simulink model "simulink_ft_fault_injection"  (R2020b)
settings: Solver=FixedStepAuto  StartTime=0.0  StopTime=Tend  FixedStep=hp  RelTol=1e-3
undefined symbols (not defined in the file): Ad_plant, Bd_plant, controller_mode, delay_length, error_probability, f, F_total, hp, K_total, mode_switching_enable, n, ref, ref_array, ref_enable, ref_sampling_factor, Sat_u, Sm
settings Model: SimulationMode=accelerator  SnapshotInterval=2  Creator=juan  LastModifiedBy=jvalencia
settings DataIOCC: ReturnWorkspaceOutputs=off
settings DebuggingCC: ArithmeticOperatorsInVariantConditions=warning
settings SFSimCC: SimUseLocalCustomCode=off  CustomCodeUndefinedFunction=UseInterfaceOnly
settings RTWCC: RTWUseLocalCustomCode=off
settings CodeAppCC: StateflowObjectComments=on

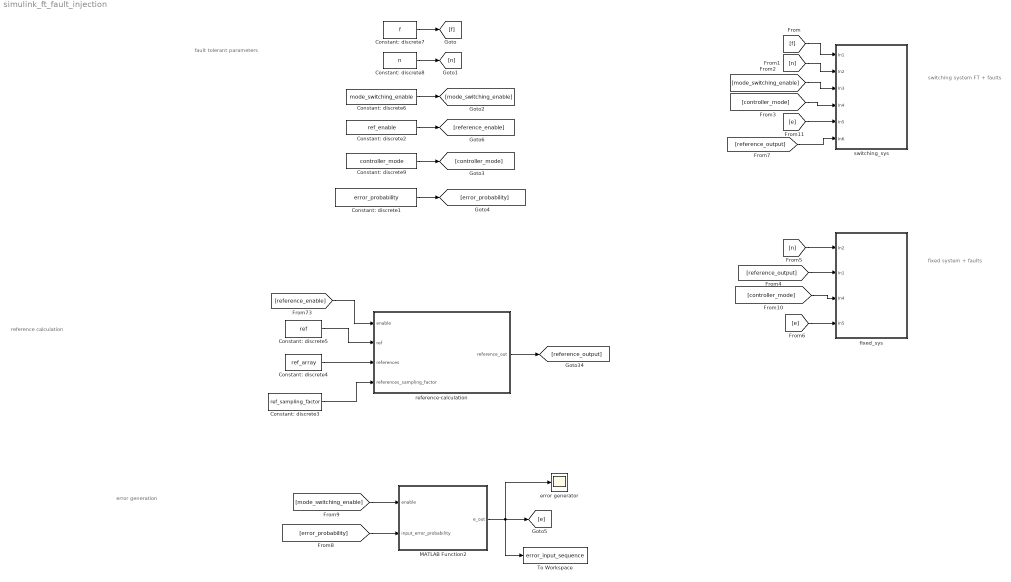
== system simulink_ft_fault_injection ==
  note: fault tolerant parameters
  note: switching system FT + faults
  note: error generation
  note: fixed system + faults
  note: reference calculation
  Constant: discrete1 : Constant  Value=error_probability  SampleTime=Sm
  Constant: discrete2 : Constant  Value=ref_enable  SampleTime=Sm
  Constant: discrete3 : Constant  Value=ref_sampling_factor  OutDataTypeStr=single  SampleTime=Sm
  Constant: discrete4 : Constant  Value=ref_array  OutDataTypeStr=single  SampleTime=Sm
  Constant: discrete5 : Constant  Value=ref  OutDataTypeStr=single  SampleTime=Sm
  Constant: discrete6 : Constant  Value=mode_switching_enable  SampleTime=Sm
  Constant: discrete7 : Constant  Value=f  OutDataTypeStr=single  SampleTime=Sm
  Constant: discrete8 : Constant  Value=n  OutDataTypeStr=single  SampleTime=Sm
  Constant: discrete9 : Constant  Value=controller_mode  SampleTime=Sm
  MATLAB Function2 : MATLAB Function  TreatAsAtomicUnit=on  SystemSampleTime=Sm
  To Workspace : ToWorkspace  VariableName=error_input_sequence  SaveFormat=Timeseries  SampleTime=Sm
  "error generator " : Scope
  fixed_sys : Subsystem
  reference-calculation : MATLAB Function  TreatAsAtomicUnit=on
  switching_sys : Subsystem
  wires:
  Constant: discrete7/1 -> [f]
  Constant: discrete8/1 -> [n]
  Constant: discrete6/1 -> [mode_switching_enable]
  Constant: discrete9/1 -> [controller_mode]
  [f] -> switching_sys/1(In1)
  [n] -> switching_sys/2(In2)
  [mode_switching_enable] -> switching_sys/3(In3)
  [controller_mode] -> switching_sys/4(In4)
  Constant: discrete1/1 -> [error_probability]
  [mode_switching_enable] -> MATLAB Function2/1(enable)
  [error_probability] -> MATLAB Function2/2(input_error_probability)
  MATLAB Function2/1(e_out) -> "error generator "/1, To Workspace/1, [e]
  [e] -> switching_sys/5(In5)
  [n] -> fixed_sys/1(In2)
  [controller_mode] -> fixed_sys/3(In4)
  [e] -> fixed_sys/4(In5)
  Constant: discrete2/1 -> [reference_enable]
  Constant: discrete4/1 -> reference-calculation/3(references)
  reference-calculation/1(reference_out) -> [reference_output]
  Constant: discrete3/1 -> reference-calculation/4(references_sampling_factor)
  Constant: discrete5/1 -> reference-calculation/2(ref)
  [reference_enable] -> reference-calculation/1(enable)
  [reference_output] -> fixed_sys/2(In1)
  [reference_output] -> switching_sys/6(In6)

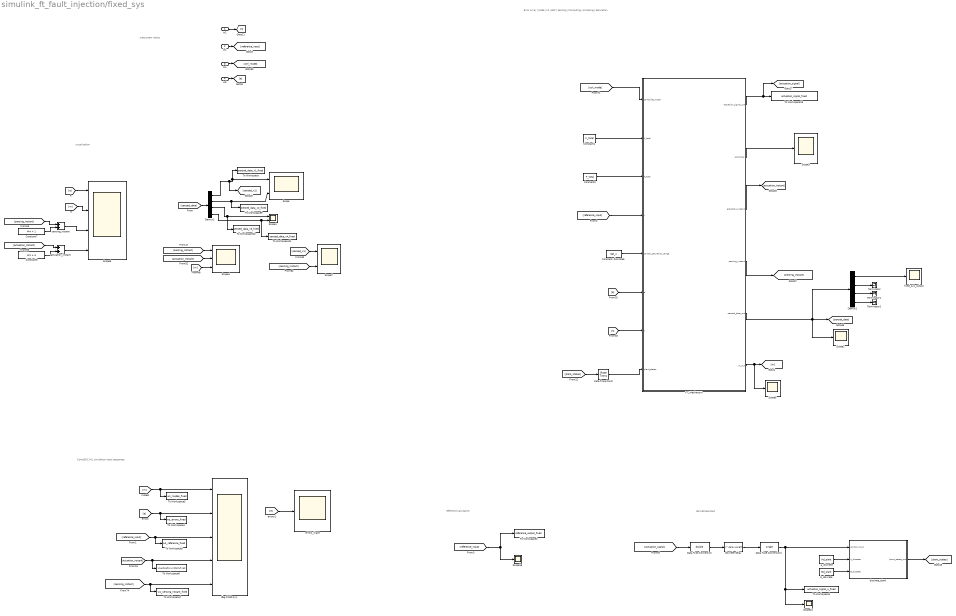
== system simulink_ft_fault_injection/fixed_sys ==
  note: Error Array | Mode | LC | EFC |
      | Sensing | Computing | Actuating | Saturation
  note: discretized plant
  note: reference calculation
  note: subsystem inputs
  note: CompSOC HIL simulation input sequences
  note: visualization
  In2 : Inport
  In1 : Inport  Port=2
  In4 : Inport  Port=3
  In5 : Inport  Port=4
  Constant1 : Constant  Value=K_total  OutDataTypeStr=single  SampleTime=Sm
  Constant2 : Constant  Value=F_total  OutDataTypeStr=single  SampleTime=Sm
  Constant7 : Constant  Value=4*n + 1  SampleTime=Sm
  Constant9 : Constant  Value=4*n + 3  SampleTime=Sm
  Constant: discrete6 : Constant  Value=Sat_u  OutDataTypeStr=single  SampleTime=Sm
  Data Type Conversion : DataTypeConversion  OutDataTypeStr=double
  Data Type Conversion1 : DataTypeConversion  OutDataTypeStr=single
  Demux1 : Demux
  Demux2 : Demux
  FT_mechanism : MATLAB Function  TreatAsAtomicUnit=on
  Rate Transition2 : RateTransition  OutPortSampleTime=Sm
  Scope : Scope  NumInputPorts=2
  Scope1 : Scope  NumInputPorts=2
  Scope{2..3,5,10,16} (5 alike) : Scope
  Scope4 : Scope  NumInputPorts=3
  Scope7 : Scope  NumInputPorts=2
  Scope9 : Scope  NumInputPorts=4
  Terminator : Terminator
  Terminator1 : Terminator
  Terminator2 : Terminator
  To Workspace : ToWorkspace  VariableName=sensed_data_x1_fixed  SaveFormat=Timeseries  SampleTime=Sm
  To Workspace1 : ToWorkspace  VariableName=actuation_signal_u_fixed  SaveFormat=Timeseries  SampleTime=Sm
  To Workspace10 : ToWorkspace  VariableName=sensed_data_x3_fixed  SaveFormat=Timeseries  SampleTime=Sm
  To Workspace11 : ToWorkspace  VariableName=sensed_data_x4_fixed  SaveFormat=Timeseries  SampleTime=Sm
  To Workspace13 : ToWorkspace  VariableName=actuation_signal_fixed  SaveFormat=Timeseries  SampleTime=Sm
  To Workspace2 : ToWorkspace  VariableName=reference_output_fixed  SaveFormat=Timeseries  SampleTime=Sm
  To Workspace3 : ToWorkspace  VariableName=ws_modes_fixed  SaveFormat=Timeseries  SampleTime=Sm
  To Workspace4 : ToWorkspace  VariableName=ws_errors_fixed  SaveFormat=Timeseries  SampleTime=Sm
  To Workspace5 : ToWorkspace  VariableName=ws_reference_fixed  SaveFormat=Timeseries  SampleTime=Sm
  To Workspace6 : ToWorkspace  VariableName=ws_actuation_instant_fixed  SaveFormat=Timeseries  SampleTime=Sm
  To Workspace7 : ToWorkspace  VariableName=ws_sensing_instant_fixed  SaveFormat=Timeseries  SampleTime=Sm
  To Workspace9 : ToWorkspace  VariableName=sensed_data_x2_fixed  SaveFormat=Timeseries  SampleTime=Sm
  a_discrete : Constant  Value=Ad_plant  OutDataTypeStr=single  SampleTime=hp
  actuation_instant : Sum
  b_discrete : Constant  Value=Bd_plant  OutDataTypeStr=single  SampleTime=hp
  dbg FIXED sys. : Scope  NumInputPorts=5
  discrete-delay : Delay  DelayLength=delay_length  SampleTime=hp
  discrete_plant : MATLAB Function  TreatAsAtomicUnit=on  SystemSampleTime=hp
  errors_trace : Scope
  "fixed_sys_output " : Scope
  sensing_instant : Sum
  wires:
  [reference_input] -> FT_mechanism/4(r)
  Demux2/1 -> [sensed_x1], To Workspace/1, Scope/1
  actuation_instant/1 -> Scope9/4
  [sensed_x1] -> Scope7/1
  discrete-delay/1 -> Data Type Conversion1/1
  [sensing_instant] -> Scope7/2
  Data Type Conversion/1 -> discrete-delay/1
  [e] -> Scope9/1
  [actuation_signal] -> Data Type Conversion/1
  [reference_input] -> To Workspace2/1, Scope16/1
  Data Type Conversion1/1 -> discrete_plant/1(control_input), To Workspace1/1, Scope10/1
  Demux2/3 -> To Workspace10/1, Scope1/1
  Demux2/4 -> To Workspace11/1, Scope1/2
  Demux2/2 -> To Workspace9/1, Scope/2
  FT_mechanism/1(actuation_signal_out) -> To Workspace13/1, [actuation_signal]
  Constant7/1 -> sensing_instant/2
  FT_mechanism/2(controller) -> Scope3/1
  [actuation_instant] -> actuation_instant/1
  Constant9/1 -> actuation_instant/2
  [sensing_instant] -> sensing_instant/1
  [actuation_instant] -> Scope4/2
  [m] -> Scope4/3
  [sensing_instant] -> Scope4/1
  [m] -> Scope9/2
  [sensed_data] -> Demux2/1
  In2/1 -> [n]
  In4/1 -> [ctrl_mode]
  In5/1 -> [e]
  [m] -> To Workspace3/1, dbg FIXED sys./1
  [reference_input] -> dbg FIXED sys./3, To Workspace5/1
  [e] -> To Workspace4/1, dbg FIXED sys./2
  [actuation_instant] -> To Workspace6/1, dbg FIXED sys./4
  [sensing_instant] -> To Workspace7/1, dbg FIXED sys./5
  a_discrete/1 -> discrete_plant/2(A_discrete)
  b_discrete/1 -> discrete_plant/3(B_discrete)
  discrete_plant/1(plant_states_out) -> [plant_states]
  Constant: discrete6/1 -> FT_mechanism/5(control_saturation_range)
  FT_mechanism/3(actuation_instant) -> [actuation_instant]
  [n] -> FT_mechanism/7(n)
  [e] -> FT_mechanism/6(e)
  Rate Transition2/1 -> FT_mechanism/8(plant_states)
  [plant_states] -> Rate Transition2/1
  FT_mechanism/5(sensed_data_out) -> Demux1/1, Scope2/1, [sensed_data]
  FT_mechanism/4(sensing_instant) -> [sensing_instant]
  [ctrl_mode] -> FT_mechanism/1(controller_mode)
  FT_mechanism/6(m_out) -> Scope5/1, [m]
  [e] -> errors_trace/1
  Demux1/1 -> "fixed_sys_output "/1
  In1/1 -> [reference_input]
  Constant1/1 -> FT_mechanism/2(K_total)
  Constant2/1 -> FT_mechanism/3(F_total)
  Demux1/2 -> Terminator/1
  Demux1/3 -> Terminator1/1
  Demux1/4 -> Terminator2/1
  sensing_instant/1 -> Scope9/3

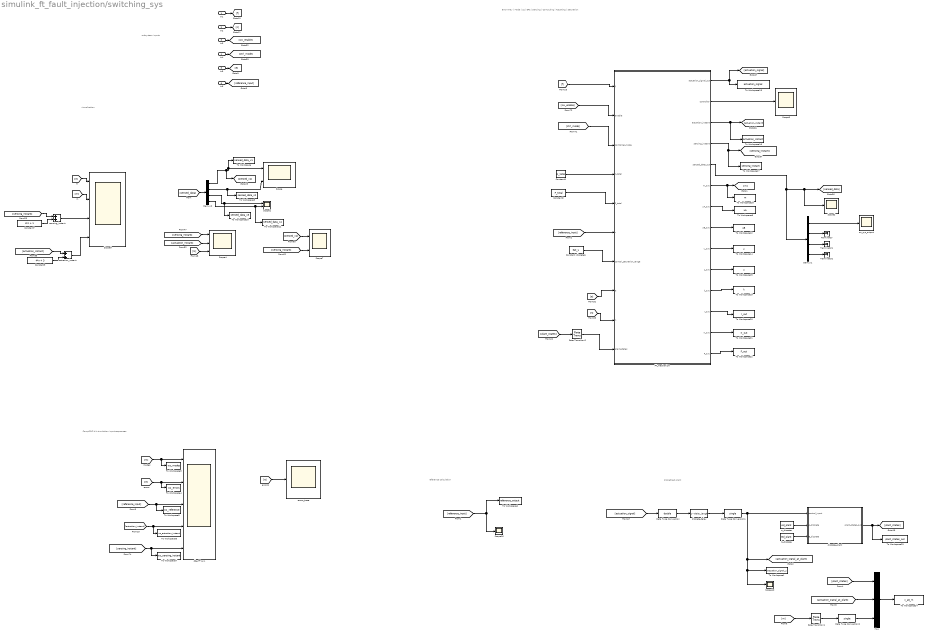
== system simulink_ft_fault_injection/switching_sys ==
  note: Error Array | Mode | LC | EFC |
      | Sensing | Computing | Actuating | Saturation
  note: discretized plant
  note: reference calculation
  note: subsystem inputs
  note: CompSOC HIL simulation input sequences
  note: visualization
  In1 : Inport
  In2 : Inport  Port=2
  In3 : Inport  Port=3
  In4 : Inport  Port=4
  In5 : Inport  Port=5
  In6 : Inport  Port=6
  Constant1 : Constant  Value=K_total  OutDataTypeStr=single  SampleTime=Sm
  Constant2 : Constant  Value=F_total  OutDataTypeStr=single  SampleTime=Sm
  Constant7 : Constant  Value=4*n + 1  SampleTime=Sm
  Constant9 : Constant  Value=4*n + 3  SampleTime=Sm
  Constant: discrete6 : Constant  Value=Sat_u  OutDataTypeStr=single  SampleTime=Sm
  Data Type Conversion : DataTypeConversion  OutDataTypeStr=double
  Data Type Conversion1 : DataTypeConversion  OutDataTypeStr=single
  Data Type Conversion2 : DataTypeConversion  OutDataTypeStr=single
  Demux1 : Demux
  Demux2 : Demux
  FT_mechanism : MATLAB Function  TreatAsAtomicUnit=on
  Mux : Mux  Inputs=3
  Rate Transition1 : RateTransition  OutPortSampleTime=hp
  Rate Transition2 : RateTransition  OutPortSampleTime=Sm
  Scope : Scope  NumInputPorts=2
  Scope1 : Scope  NumInputPorts=2
  Scope{2..3,10,16} (4 alike) : Scope
  Scope4 : Scope  NumInputPorts=3
  Scope7 : Scope  NumInputPorts=2
  Scope9 : Scope  NumInputPorts=4
  Terminator : Terminator
  Terminator1 : Terminator
  Terminator2 : Terminator
  To Workspace : ToWorkspace  VariableName=sensed_data_x1  SaveFormat=Timeseries  SampleTime=Sm
  To Workspace1 : ToWorkspace  VariableName=actuation_signal_u  SaveFormat=Timeseries  SampleTime=Sm
  To Workspace10 : ToWorkspace  VariableName=sensed_data_x3  SaveFormat=Timeseries  SampleTime=Sm
  To Workspace11 : ToWorkspace  VariableName=sensed_data_x4  SaveFormat=Timeseries  SampleTime=Sm
  To Workspace12 : ToWorkspace  VariableName=uB  SaveFormat=Timeseries  SampleTime=Sm
  To Workspace13 : ToWorkspace  VariableName=actuation_signal  SaveFormat=Timeseries  SampleTime=Sm
  To Workspace14 : ToWorkspace  VariableName=u  SaveFormat=Timeseries  SampleTime=Sm
  To Workspace15 : ToWorkspace  VariableName=z  SaveFormat=Timeseries  SampleTime=-1
  To Workspace16 : ToWorkspace  VariableName=actuation_instant  SaveFormat=Timeseries  SampleTime=Sm
  To Workspace17 : ToWorkspace  VariableName=sensing_instant  SaveFormat=Timeseries  SampleTime=Sm
  To Workspace18 : ToWorkspace  VariableName=m  SaveFormat=Timeseries  SampleTime=Sm
  To Workspace19 : ToWorkspace  VariableName=k  SaveFormat=Timeseries  SampleTime=Sm
  To Workspace2 : ToWorkspace  VariableName=reference_output  SaveFormat=Timeseries  SampleTime=Sm
  To Workspace20 : ToWorkspace  VariableName=r_out  SaveFormat=Timeseries  SampleTime=Sm
  To Workspace21 : ToWorkspace  VariableName=K_out  SaveFormat=Timeseries  SampleTime=Sm
  To Workspace22 : ToWorkspace  VariableName=F_out  SaveFormat=Timeseries  SampleTime=Sm
  To Workspace23 : ToWorkspace  VariableName=plant_states_out  SaveFormat=Timeseries  SampleTime=hp
  To Workspace24 : ToWorkspace  VariableName=x_aS_m  SaveFormat=Timeseries  SampleTime=hp
  To Workspace3 : ToWorkspace  VariableName=ws_modes  SaveFormat=Timeseries  SampleTime=Sm
  To Workspace4 : ToWorkspace  VariableName=ws_errors  SaveFormat=Timeseries  SampleTime=Sm
  To Workspace5 : ToWorkspace  VariableName=ws_reference  SaveFormat=Timeseries  SampleTime=Sm
  To Workspace6 : ToWorkspace  VariableName=ws_actuation_instant  SaveFormat=Timeseries  SampleTime=Sm
  To Workspace7 : ToWorkspace  VariableName=ws_sensing_instant  SaveFormat=Timeseries  SampleTime=Sm
  To Workspace8 : ToWorkspace  VariableName=uA  SaveFormat=Timeseries  SampleTime=Sm
  To Workspace9 : ToWorkspace  VariableName=sensed_data_x2  SaveFormat=Timeseries  SampleTime=Sm
  a_discrete : Constant  Value=Ad_plant  OutDataTypeStr=single  SampleTime=hp
  actuation_instant : Sum
  b_discrete : Constant  Value=Bd_plant  OutDataTypeStr=single  SampleTime=hp
  dbg FT sys. : Scope  NumInputPorts=5
  discrete-delay : Delay  DelayLength=delay_length  SampleTime=hp
  discrete_plant : MATLAB Function  TreatAsAtomicUnit=on  SystemSampleTime=hp
  errors_trace : Scope
  sensing_instant : Sum
  sw_sys_output : Scope
  wires:
  [reference_input] -> FT_mechanism/6(r)
  Demux2/1 -> [sensed_x1], To Workspace/1, Scope/1
  actuation_instant/1 -> Scope9/4
  [sensed_x1] -> Scope7/1
  discrete-delay/1 -> Data Type Conversion1/1
  [sensing_instant] -> Scope7/2
  Data Type Conversion/1 -> discrete-delay/1
  [e] -> Scope9/1
  [actuation_signal] -> Data Type Conversion/1
  [reference_input] -> To Workspace2/1, Scope16/1
  Data Type Conversion1/1 -> discrete_plant/1(control_input), To Workspace1/1, Scope10/1, [actuation_signal_at_plant]
  Demux2/3 -> To Workspace10/1, Scope1/1
  Demux2/4 -> To Workspace11/1, Scope1/2
  Demux2/2 -> To Workspace9/1, Scope/2
  FT_mechanism/1(actuation_signal_out) -> To Workspace13/1, [actuation_signal]
  Constant7/1 -> sensing_instant/2
  FT_mechanism/2(controller) -> Scope3/1
  [actuation_instant] -> actuation_instant/1
  Constant9/1 -> actuation_instant/2
  [sensing_instant] -> sensing_instant/1
  [actuation_instant] -> Scope4/2
  [m] -> Scope4/3
  [sensing_instant] -> Scope4/1
  [m] -> Scope9/2
  [sensed_data] -> Demux2/1
  In1/1 -> [f]
  In2/1 -> [n]
  In3/1 -> [sw_enable]
  In4/1 -> [ctrl_mode]
  In5/1 -> [e]
  [m] -> To Workspace3/1, dbg FT sys./1
  [reference_input] -> dbg FT sys./3, To Workspace5/1
  [e] -> To Workspace4/1, dbg FT sys./2
  [actuation_instant] -> To Workspace6/1, dbg FT sys./4
  [sensing_instant] -> To Workspace7/1, dbg FT sys./5
  a_discrete/1 -> discrete_plant/2(A_discrete)
  b_discrete/1 -> discrete_plant/3(B_discrete)
  discrete_plant/1(plant_states_out) -> To Workspace23/1, [plant_states]
  Constant: discrete6/1 -> FT_mechanism/7(control_saturation_range)
  FT_mechanism/3(actuation_instant) -> To Workspace16/1, [actuation_instant]
  [n] -> FT_mechanism/9(n)
  [e] -> FT_mechanism/8(e)
  Rate Transition2/1 -> FT_mechanism/10(plant_states)
  [plant_states] -> Rate Transition2/1
  FT_mechanism/5(sensed_data_out) -> Demux1/1, Scope2/1, [sensed_data]
  FT_mechanism/4(sensing_instant) -> To Workspace17/1, [sensing_instant]
  [sw_enable] -> FT_mechanism/2(enable)
  [ctrl_mode] -> FT_mechanism/3(controller_mode)
  [f] -> FT_mechanism/1(f)
  FT_mechanism/6(m_out) -> To Workspace18/1, [m]
  [e] -> errors_trace/1
  Demux1/1 -> sw_sys_output/1
  In6/1 -> [reference_input]
  Constant1/1 -> FT_mechanism/4(K_total)
  Constant2/1 -> FT_mechanism/5(F_total)
  Demux1/2 -> Terminator/1
  Demux1/3 -> Terminator1/1
  Demux1/4 -> Terminator2/1
  sensing_instant/1 -> Scope9/3
  FT_mechanism/7(uA_out) -> To Workspace8/1
  FT_mechanism/9(u_out) -> To Workspace14/1
  FT_mechanism/8(uB_out) -> To Workspace12/1
  FT_mechanism/10(z_out) -> To Workspace15/1
  FT_mechanism/11(k_out) -> To Workspace19/1
  FT_mechanism/12(r_out) -> To Workspace20/1
  FT_mechanism/13(K_out) -> To Workspace21/1
  FT_mechanism/14(F_out) -> To Workspace22/1
  [plant_states] -> Mux/1
  [actuation_signal_at_plant] -> Mux/2
  Mux/1 -> To Workspace24/1
  [m] -> Rate Transition1/1
  Data Type Conversion2/1 -> Mux/3
  Rate Transition1/1 -> Data Type Conversion2/1

== matlab function simulink_ft_fault_injection/MATLAB Function2 ==
  data: e_out output; enable input; input_error_probability input
function e_out = error_generation(enable, input_error_probability)

persistent execution_counter;
if (isempty(execution_counter)) %It does not already exist
execution_counter = 1; % initialize with 1
end

persistent counter;
if (isempty(counter)) %It does not already exist
counter = 1; % initialize with 1
end

%% test sequence: c1 since there are no errors
sequence = 0; 

if ( counter == length(sequence) )
    counter = 1;
else
    counter = counter + 1;
end

e = sequence(counter);


%% test random error
error_probability = input_error_probability;

if (execution_counter < 5000 )
    error_probability_temp = error_probability(1);
else
    error_probability_temp = error_probability(2);
end

temp = unifrnd(0,1);
if (temp > (1-error_probability_temp))
    e = 1;
else
    e = 0;
end


%% enable error injection in the simulation
if enable == 1
    e_out = e;
else
    e_out = 0;
end

%% increase execution counter
execution_counter = execution_counter + 1;

== matlab function simulink_ft_fault_injection/fixed_sys/FT_mechanism ==
  data: controller_mode input; K_total input; F_total input; r input single; control_saturation_range input; e input; n input; actuation_signal_out output single; controller output; actuation_instant output; sensing_instant output; plant_states input single size=4; sensed_data_out output single size=4; m_out output
function [actuation_signal_out, controller, actuation_instant, sensing_instant, sensed_data_out, m_out] = computing(controller_mode, K_total, F_total, r, control_saturation_range, e, n, plant_states)
% deleted output
% error_free_counter_out

%% initialization of persistent variables
%#eml
assert(n < 20); % less than 10 modes: limit for embedded code this can be changed

% error array
persistent e_array;
if (isempty(e_array)) %It does not already exist
    e_array = zeros(1,2^(n+1)); % initialize with 0
end

% mode
persistent m;
if (isempty(m)) %It does not already exist
    m = 1; % initialize with mode 1
end

% current mode
persistent current_mode;
if (isempty(current_mode)) %It does not already exist
    current_mode = 1; % initialize with mode 1
end

% lc
persistent location_counter;
if (isempty(location_counter)) %It does not already exist
    location_counter = 0; % initialize with 0
end

persistent lc_old;
if (isempty(lc_old)) %It does not already exist
    lc_old = 0; % initialize with 0
end


% efc
persistent error_free_counter;
if (isempty(error_free_counter)) %It does not already exist
    error_free_counter = zeros(n,1); % initialize with 0. TODO: fixed 3 = n generic coding
end

% u
persistent u;
if (isempty(u)) %It does not already exist
    u = single(0); % initialize with 0.
end

persistent old_u;
if (isempty(old_u)) %It does not already exist
    old_u = single(0); % initialize with 0.
end

% actuation_signal
persistent actuation_signal;
if (isempty(actuation_signal)) %It does not already exist
    actuation_signal = single(0); % initialize with 0.
end

persistent old_actuation_signal;
if (isempty(old_actuation_signal)) %It does not already exist
    old_actuation_signal = single(0); % initialize with 0.
end



%% error array update
% updating array
for i = 1:2^(n+1)
    if ( i < 2^(n+1) )
        e_array(i) = e_array(i+1);
    else
        e_array(i) = e; 
    end
end



%% m_out
% setting a fixed mode: here we can set a mode for testings
current_mode = controller_mode;
m            = current_mode;
m_out        = m; % fixed mode within the script



%% function location_counter_out = location_counter_calculation(m, current_mode, old_location_counter)
if ( location_counter >= 2^(current_mode+1) )
    location_counter = 1;
else
    if ( location_counter >= 2^(m+1) )
        location_counter = 1;
    else
        location_counter = lc_old +1;
    end
end



%% function error_free_counter_out  = error_free_counter_calculation(e, n, m, location_counter, old_error_free_counter)
% main algorithm
if (location_counter >= 2^(m+1))
    for i = 1:n
        if ( i ~= m )
            error_free_counter(i) = 0;
        else            
            if( sum(e_array(2^n-2^i+1:2^n)) < 2^i-1 )
                error_free_counter(i) = error_free_counter(i) + 1;
            else
                error_free_counter(i) = 0;
            end          
        end
    end
       
else
    for i = 1:n
        if ( i ~= m )
            error_free_counter(i) = 0;
        else
            error_free_counter(i) = error_free_counter(i);
        end
    end    

end

error_free_counter_out = error_free_counter;





%% function [sensed_data_out,sensing_instant] = sensing(location_counter, old_sensed_data, plant_states)
persistent sensed_data;
if (isempty(sensed_data)) %It does not already exist
    sensed_data = single(ones(4,1)); % initialize with 0. TODO: make generic 4 = dimension
end

persistent z;
if (isempty(z)) %It does not already exist
    z = single(ones(5,1)); % initialize with 0. TODO: make generic 4 = dimension
end

if ( location_counter == 1 )
    sensed_data = plant_states; 
    z = [sensed_data; old_u];
    
    sensing_instant = 1;
else
    sensed_data = sensed_data; 
    z = z;    
    
    sensing_instant = 0;
end

sensed_data_out =  sensed_data;




%% computation
for i = 1:m
   u = K_total(i,:)*z + F_total(i)*r;   
end
controller = m;



%% function [actuation_signal_out,actuation_instant] = actuating(e, n, m, location_counter, control_input, old_actuation_signal)
% main algorithm
if ( location_counter == 2^(m+1) )
    if( sum(e_array(2^(n+1)-2^(m+1)+1:2^(n+1))) >= 2^(m+1)-1 )        
        actuation_signal = old_actuation_signal; % fault effect (use old sample)
%         actuation_signal = single(0); % fault effect (zero the actuation signal)
    else
        actuation_signal = u;
    end        
    actuation_instant = 1;
else
    actuation_instant = 0;
end




%% saturation
actuation_signal_out = actuation_signal;


%% update old signals
current_mode         = m;
lc_old               = location_counter;
old_actuation_signal = actuation_signal;
old_u                = u;

== matlab function simulink_ft_fault_injection/fixed_sys/discrete_plant ==
  data: control_input input single; plant_states_out output single; A_discrete input single; B_discrete input single
function plant_states_out = discrete_plant(control_input, A_discrete, B_discrete)

persistent state;
if (isempty(state)) %It does not already exist
state = single(ones(4,1)); % initialize with 0
end

plant_states_out = A_discrete*state + B_discrete*control_input;
state = single(plant_states_out);

== matlab function simulink_ft_fault_injection/switching_sys/discrete_plant ==
  data: control_input input single; plant_states_out output single; A_discrete input single; B_discrete input single
function plant_states_out = discrete_plant(control_input, A_discrete, B_discrete)

persistent state;
if (isempty(state)) %It does not already exist
state = single(zeros(4,1)); % initialize with 0
end

plant_states_out = A_discrete*state + B_discrete*control_input;
state = single(plant_states_out);

== matlab function simulink_ft_fault_injection/reference-calculation ==
  data: enable input; ref input; references input; reference_out output; references_sampling_factor input
function reference_out = input_reference(enable, ref, references, references_sampling_factor)
%% VARIABLE DECLARATIONS OF COUNTERS
persistent reference_counter;
if (isempty(reference_counter)) %It does not already exist
    reference_counter = 1; % initialize with mode 1
end

persistent sampling_counter;
if (isempty(sampling_counter)) %It does not already exist
    sampling_counter = 1; % initialize with mode 1
end

%% READING INPUT VARIABLES TEMPORALLY
ref_temp        = ref;
references_temp = references;

%% OUTPUT
if enable == 1
    reference_out = single(references_temp(reference_counter));
else
    reference_out = single(ref_temp);
end

% reference_out = single(0); % stability test

%% updating the sampling counter
if sampling_counter == references_sampling_factor
    sampling_counter = 1;
else
    sampling_counter = sampling_counter + 1;
end

%% updating the reference counter to select a different reference
if sampling_counter == 1
    if reference_counter < length(references_temp)
        reference_counter = reference_counter + 1;
    else
        reference_counter = 1;
    end
end

== matlab function simulink_ft_fault_injection/switching_sys/FT_mechanism ==
  data: f input; enable input; controller_mode input; K_total input; F_total input; r input single; control_saturation_range input; e input; n input; actuation_signal_out output single; controller output; actuation_instant output; sensing_instant output; plant_states input single size=4; sensed_data_out output single size=4; m_out output; uA_out output; uB_out output; u_out output; z_out output; k_out output; r_out output; K_out output; F_out output
function [actuation_signal_out, controller, actuation_instant, sensing_instant, sensed_data_out, m_out, uA_out, uB_out, u_out, z_out, k_out, r_out, K_out, F_out] = computing(f, enable, controller_mode, K_total, F_total, r, control_saturation_range, e, n, plant_states)
% deleted outputs:
% error_free_counter_out

%% initialization of persistent variables
%#eml
assert(n < 20); % less than 10 modes: limit for embedded code this can be changed

% error array
persistent e_array;
if (isempty(e_array)) %It does not already exist
    e_array = zeros(1,2^(n+1)); % initialize with 0
end

% u array
persistent u_array;
if (isempty(u_array)) %It does not already exist
    u_array = zeros(1,2^(n+1)); % initialize with 0
end

% k
persistent k;
if (isempty(k)) %It does not already exist
    k = 0; % initialize with k=0
end

% mode
persistent m;
if (isempty(m)) %It does not already exist
    m = 1; % initialize with mode 1
end

% current mode
persistent current_mode;
if (isempty(current_mode)) %It does not already exist
    current_mode = 1; % initialize with mode 1
end

% lc
persistent location_counter;
if (isempty(location_counter)) %It does not already exist
    location_counter = 0; % initialize with 0
end

persistent lc_old;
if (isempty(lc_old)) %It does not already exist
    lc_old = 0; % initialize with 0
end


% efc
persistent error_free_counter;
if (isempty(error_free_counter)) %It does not already exist
    error_free_counter = zeros(n,1); % initialize with 0. TODO: fixed 3 = n generic coding
end

% uA
persistent uA;
if (isempty(uA)) %It does not already exist
    uA = single(0); % initialize with 0.
end

% uB
persistent uB;
if (isempty(uB)) %It does not already exist
    uB = single(0); % initialize with 0.
end

% u
persistent u;
if (isempty(u)) %It does not already exist
    u = single(0); % initialize with 0.
end

persistent old_u;
if (isempty(old_u)) %It does not already exist
    old_u = single(0); % initialize with 0.
end

% actuation_signal
persistent actuation_signal;
if (isempty(actuation_signal)) %It does not already exist
    actuation_signal = single(0); % initialize with 0.
end

% old_actuation_signal
persistent old_actuation_signal;
if (isempty(old_actuation_signal)) %It does not already exist
    old_actuation_signal = single(0); % initialize with 0.
end




%% error array update
% updating array
for i = 1:2^(n+1)
    if ( i < 2^(n+1) )
        e_array(i) = e_array(i+1);
    else
        e_array(i) = e; 
    end
end



%% function m_out = mode_calculation(e, f, old_error_free_counter, n, old_m, enable, controller_mode)
% algorithm
if(current_mode < n)
    for i = 1:n
        if( current_mode == i )
            if( sum(e_array(2^(n+1)-2^(i+1)+1:2^(n+1))) >= 2^(i+1)-1 )
                if( error_free_counter(i) >= f(i) )
                    m = current_mode + 1;
                else
                    m = current_mode;
                end
            else
                if( error_free_counter(i) >= f(i) )
                    if ( current_mode > 1)
                        m = current_mode - 1;
                    else
                        m = current_mode;
                    end
                else
                    m = current_mode;
                end                                    
            end            
        end
    end
else
    for i = 1:n
        if( current_mode == i )
            if( error_free_counter(i) >= f(i) )
                m = current_mode - 1;
            else
                m = current_mode;
            end    
        end
    end
end


% USING THE ENABLE SIGNAL: ASSIGNING CONSTANT MODE IF SW IS NOT ENABLED
if enable == 1
    m_out = m;
else
    current_mode = controller_mode;
    m            = current_mode;
    m_out        = m; % fixed mode within the script
end


























%% function location_counter_out = location_counter_calculation(m, current_mode, old_location_counter)
if ( location_counter >= 2^(current_mode+1) )
    location_counter = 1;
else
    if ( location_counter >= 2^(m+1) )
        location_counter = 1;
    else
        location_counter = lc_old +1;
    end
end



%% function error_free_counter_out  = error_free_counter_calculation(e, n, m, location_counter, old_error_free_counter)
% main algorithm
if (location_counter >= 2^(m+1))
    for i = 1:n
        if ( i ~= m )
            error_free_counter(i) = 0;
        else            
            if( sum(e_array(2^(n+1)-2^(i+1)+1:2^(n+1))) < 2^(i+1)-1 )
                error_free_counter(i) = error_free_counter(i) + 1;
            else
                error_free_counter(i) = 0;
            end          
        end
    end
       
else
    for i = 1:n
        if ( i ~= m )
            error_free_counter(i) = 0;
        else
            error_free_counter(i) = error_free_counter(i);
        end
    end    

end

error_free_counter_out = error_free_counter;





%% function [sensed_data_out,sensing_instant] = sensing(location_counter, old_sensed_data, plant_states)
persistent sensed_data;
if (isempty(sensed_data)) %It does not already exist
    sensed_data = single(zeros(4,1)); % initialize with 0. TODO: make generic 4 = dimension
end

persistent z;
if (isempty(z)) %It does not already exist
    z = single(zeros(5,1)); % initialize with 0. TODO: make generic 4 = dimension
end

if ( location_counter == 1 )
    sensed_data = plant_states; 
%     z = [sensed_data; old_u];
    z = [sensed_data; old_actuation_signal];
    
    sensing_instant = 1;
else
    sensed_data = sensed_data; 
    z = z;    
    
    sensing_instant = 0;
end


sensed_data_out =  sensed_data;
z_out = z;

%% computation
% % working code as per 14.06.2021 --------------------
% K = K_total(m,:);
% F = F_total(m);
% 
% uA = K*z;
% uB = F*r;
% u = uA + uB;   
% 
% uA_out = uA;
% uB_out = uB;
% u_out  = u;
% 
% controller = m;
% % ---------------------------------------------------

% getting right K, F function of (m)
K = K_total(m,:);
F = F_total(m);

% computing feedback and feedforward parts
uA = K*z;
uB = F*r;
u = uA + uB;   
   
% u array update: u_array of size 2^{n+1) load the new u into the array
for i = 1:2^(n+1)
    if ( i < 2^(n+1) )
        u_array(i) = u_array(i+1);
    else
        u_array(i) = u; 
    end
end



%% output values [for debugging]
uA_out = uA;
uB_out = uB;
u_out  = u;

controller = m;



%% function [actuation_signal_out,actuation_instant] = actuating(e, n, m, location_counter, control_input, old_actuation_signal)
% main algorithm
if ( location_counter == 2^(m+1) )
    % actuation instant flag
    actuation_instant = 1;
    
    % selection of u among elements of u_array depending of the error_array
    temp_error_array = e_array(2^(n+1)-2^(m+1)+1 : 2^(n+1));
    temp_u_array     = u_array(2^(n+1)-2^(m+1)+1 : 2^(n+1));

    not_e_array = not(temp_error_array);
    not_e_array_shift_left_with_0 = [not_e_array(2:end) 0];
    u_shiftleft = not_e_array_shift_left_with_0 .* temp_u_array;
        
    
    [is_there_1, where_is_first_1] =  ismember(1, flip( not_e_array_shift_left_with_0 ));
    if is_there_1 == 1
        location_last_correct_computation = 1 + length(not_e_array_shift_left_with_0) - where_is_first_1;
    else 
        location_last_correct_computation = 1; % all values are 0 
    end
    
    
%     location_last_correct_computation = find(not_e_array_shift_left_with_0, 1, 'last');
    last_correct_computation = single( u_shiftleft(location_last_correct_computation) );
    
        
    if all(u_shiftleft == 0) % vector is full of zeros 
        u = single( sum(u_shiftleft) ); % sum of zeros       
    else
        u = single( last_correct_computation ); % find last correct computation
    end
          
    
    if( sum(e_array(2^(n+1)-2^(m+1)+1:2^(n+1))) >= 2^(m+1)-1 )
        actuation_signal = old_actuation_signal; % fault effect (use old sample) 
    else
        actuation_signal = u;
    end       
    
else
    % actuation instant flag
    actuation_instant = 0;
    
end




%% saturation
actuation_signal_out = actuation_signal;

%% k
k_out=k;

%% r
r_out=r;

%% F
F_out = F;

%% K
K_out = K;


%% update old signals
current_mode = m;
lc_old = location_counter;
old_actuation_signal = actuation_signal;
old_u = u;
k=k+1;
